simulink model "DC_Motor_Simulation"  (R2025a)
settings: Solver=ode23tb  StartTime=0.0  StopTime=10.0  MaxStep=1e-4  RelTol=1e-3
libraries: spsDCVoltageSourceLib x2, spsDCMachineLib x1, sps_lib x1
settings Model: Creator=Jawad  LastModifiedBy=Jawad

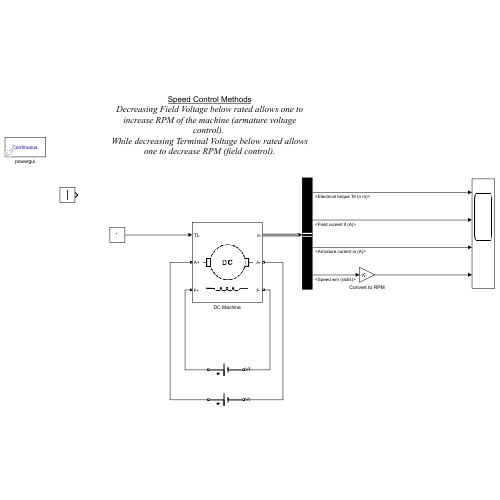
[thumbnail: Simulink's stored preview of the top-level diagram]
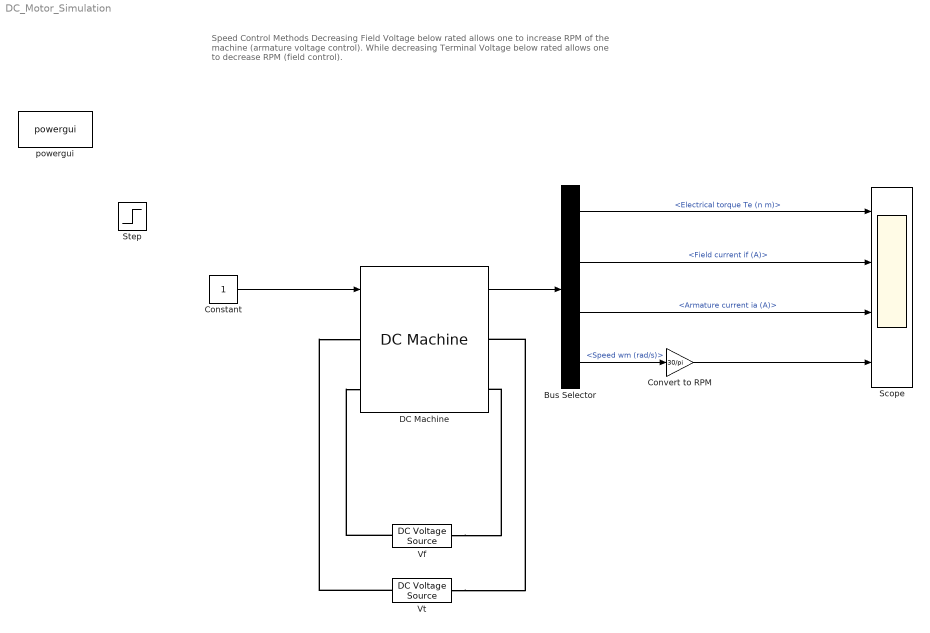
== system DC_Motor_Simulation ==
  note: Speed Control Methods
      | Decreasing Field Voltage below rated allows one to increase RPM of the machine (armature voltage control).
      | While decreasing Terminal Voltage below rated allows one to decrease RPM (field control).
  Bus Selector : BusSelector  OutputSignals=Electrical torque Te (n m),Field current if (A),Armature current ia (A),Speed wm (rad/s)
  Constant : Constant
  Convert to RPM : Gain  Gain=30/pi
  DC Machine : spsDCMachineLib/DC Machine  PresetModel=No  MechanicalLoad=Torque TL  FieldType=Wound  ShowDetailedParameters=on  MeasurementBus=off  RLa="[ 0.6  0.012]"  RLf="[ 240  120]"  Laf=1.5  MachineConstant=Torque constant (N.m/A)  Ke=1.8  Kt=1.8  J=1  Bm=0  Tf=0  w0=1  Ifinit=0.625  TsPowergui=0  TsBlock=-1
  Scope : Scope  NumInputPorts=4
      settings: ActiveDisplayYMinimum=-45.748230002523911  ActiveDisplayYMaximum=421.73512916702305
  Step : Step  Time=5  Before=1  After=100  SampleTime=0
  Vf : spsDCVoltageSourceLib/DC Voltage Source  Amplitude=150  Measurements=None
  Vt : spsDCVoltageSourceLib/DC Voltage Source  Amplitude=240  Measurements=None
  powergui : sps_lib/powergui  Priority=1  SimulationMode=Continuous  SampleTime=50e-6  frequency=60  Iterations=50  frequencyindice=0  Pbase=100e6  ErrMax=1e-4  UnitsV=kV  UnitsW=MW  buscounter=0  FunctionMessages=off  echomessages=off  EnableUseOfTLC=off  CurrentSourceSwitches=off  DisableSnubberDevices=off  DisableRonSwitches=off  DisableVfSwitches=off  DisplayEquations=off  AutomaticDiscreteSolvers=off  SolverType=Tustin/Backward Euler (TBE)  Interpol=off  ExternalGateDelay=off  methode=off  Ts=100  x0status=blocks  SPID=on  SwTol=0  HookPort=off  NonlinearTolerance=1e-4  nMaxIteration=100  ContinueOnMaxIteration=off  RestoreLinks=warning  ResistiveCurrentMeasurement=off  Frange=[0:2:500]  Ylog=off  Xlog=on  ShowGrid=off  save=off  variable=ZData  structure=0  ZoomFFT=off  StartTime=0.0  cycles=1  DisplayStyle=1  fundamental=60  FreqAxis=off  MaxFrequency=1000  frequencyindicesteady=1  RmsSteady=1  display=off
  wires:
  DC Machine/1 -> Bus Selector/1
  Bus Selector/1 -> Scope/1  "<Electrical torque Te (n m)>"
  Bus Selector/2 -> Scope/2  "<Field current if (A)>"
  Bus Selector/3 -> Scope/3  "<Armature current ia (A)>"
  Bus Selector/4 -> Convert to RPM/1  "<Speed wm (rad/s)>"
  Convert to RPM/1 -> Scope/4
  Constant/1 -> DC Machine/1
  connections:
  Vt/RConn1 -- DC Machine/LConn1
  Vt/LConn1 -- DC Machine/RConn1
  Vf/LConn1 -- DC Machine/RConn2
  Vf/RConn1 -- DC Machine/LConn2
